simulink model "observer"  (R2015a)
settings: Solver=FixedStepDiscrete  StartTime=0.0  StopTime=10.0  RelTol=1e-3
values from neighbouring files (symbols this model uses):
  A = [3.29698189006 1 0 0 -4.20791026518 0 1 0 2.48348543348 0 0 1 ... (16 elements, 4x4)]    [end_of_class.mat]    (also in log_observer_test.mat; parameters.mat)
  B = [1 0 0 0]    [end_of_class.mat]    (also in log_observer_test.mat; parameters.mat)
  C = [-0.0495309545297 0.081302844811 0.0308276179144 0]    [end_of_class.mat]    (also in log_observer_test.mat; parameters.mat)
  M = dlqe(A, G, C, Qw, Rw)    [compute_gain.m]    (also in end_of_class.mat = [46.1937797554 31.7894394899 18.6722805315 9.22195693924]; log_observer_test.mat = [13.0934534825 11.0057014889 8.5354108434 5.97963050629])
settings Model: Creator=alunos  LastModifiedBy=alunos
settings DataIOCC: LimitDataPoints=off

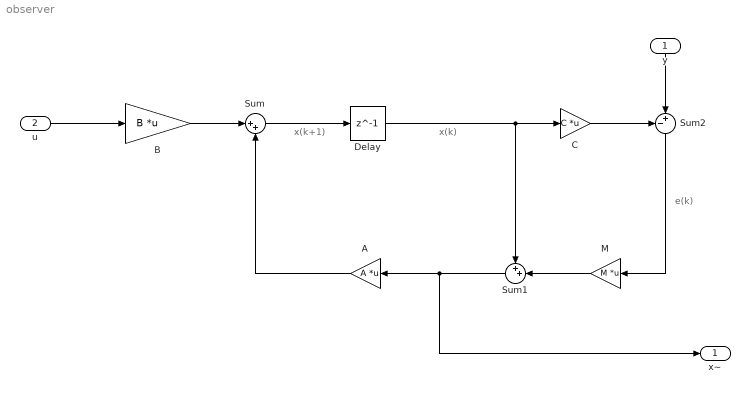
== system observer ==
  note: e(k)
  note: x(k)
  note: x(k+1)
  y : Inport  PortDimensions=1
  u : Inport  Port=2
  A : Gain  Gain=A  Multiplication=Matrix(K*u)
  B : Gain  Gain=B  Multiplication=Matrix(K*u) (u vector)
  C : Gain  Gain=C  Multiplication=Matrix(K*u)
  Delay : Delay  DelayLength=1  InitialCondition=[0;0;0;0]
  M : Gain  Gain=M  Multiplication=Matrix(K*u) (u vector)
  Sum : Sum  Inputs=|++
  Sum1 : Sum  Inputs=++|
  Sum2 : Sum  Inputs=-+|
  x~ : Outport  PortDimensions=[4,1]
  wires:
  Sum/1 -> Delay/1
  C/1 -> Sum2/1
  Sum2/1 -> M/1
  Delay/1 -> C/1, Sum1/1
  M/1 -> Sum1/2
  A/1 -> Sum/2
  y/1 -> Sum2/2
  u/1 -> B/1
  Sum1/1 -> x~/1, A/1
  B/1 -> Sum/1
